simulink model "vertical_smm_3d_with_xz_lqr_with_torque_cmds"  (R2015a)
settings: Solver=FixedStepDiscrete  SolverMode=SingleTasking  StartTime=0.0  StopTime=inf  FixedStep=sample_time  RelTol=1e-3
values from neighbouring files (symbols this model uses):
  forward_dx_of_dxstar = [-1.33147741515 -1.28147741462 -1.23147741409 -1.18147741356 -1.13147741303 -1.0814774125 -1.03147741197 -0.981477411445 -0.931477410916 -0.881477410388 -0.831477409975 -0.781477409737 ... (28413 elements, 41x21x33)]    [ref_trajs.mat]
  forward_x_of_dxstar = [0.245075236011 0.237749717983 0.230424199955 0.223098681927 0.215773163898 0.20844764587 0.201122127842 0.193796609813 0.186471091785 0.179145573757 0.171820055745 0.164494537786 ... (28413 elements, 41x21x33)]    [ref_trajs.mat]
  target_dx_range = [-1 -0.95 -0.9 -0.85 -0.8 -0.75 -0.7 -0.65 -0.6 -0.55 -0.5 -0.45 ... (41 elements, 1x41)]    [ref_trajs.mat]
undefined symbols (not defined in the file or in its folder): A_kalman_fourbar_gear, A_kalman_transverse, A_kalman_vertical, A_lpf_accelerometer, A_lpf_dtau, A_lpf_fourbar_angles, A_lpf_imu, A_lpf_lateral_angle, A_lpf_leg_spring, B1_lpf_accelerometer, B1_lpf_dtau, B1_lpf_fourbar_angles, B1_lpf_imu, B1_lpf_lateral_angle, B1_lpf_leg_spring, B2_lpf_accelerometer, B2_lpf_dtau, B2_lpf_fourbar_angles, B2_lpf_imu, B2_lpf_lateral_angle, B2_lpf_leg_spring, B_dx_versus_x0, B_kalman_fourbar_gear, B_kalman_transverse, B_kalman_vertical, backwards_K_sag_of_t, backwards_P_sag_of_t, C_kalman_fourbar_gear, C_kalman_transverse, C_kalman_vertical, com_leg_motor, com_torso, contact_threshold, control_start_time, d_ankle_to_foot, d_vertical_com, desired_com_forward_velocity, desired_com_lateral_velocity, desired_initial_leg_roll_left, desired_initial_leg_roll_right, desired_stance_beta2, desired_standing_torso_pitch, desired_standing_torso_roll, desired_standing_z, desired_torso_pitch, desired_torso_roll, Discrete, enable_bouncing, enable_hopping, fcut_contact, g, HIP_MTR_MAX_CONT_TORQUE, HIP_MTR_MAX_TORQUE, i_leg_motor, i_robot, i_torso, initial_dx_estimate, initial_dy_estimate, initial_dz_estimate, initial_leg_selection ... (+77)
libraries: simulink x18, ctrlSharedLib x7
(part 2 of 5)

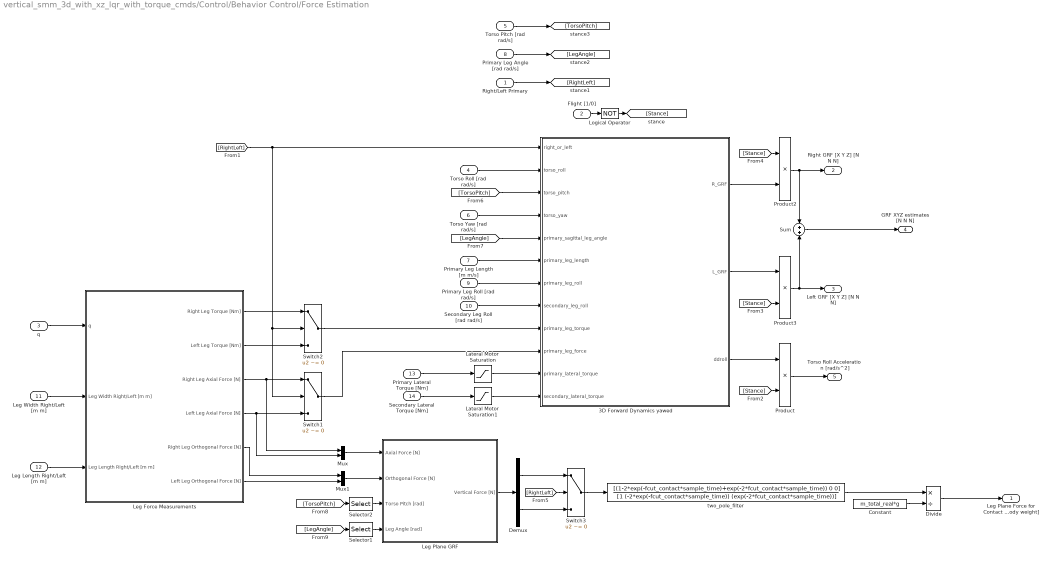
== system vertical_smm_3d_with_xz_lqr_with_torque_cmds/Control/Behavior Control/Force Estimation ==
  Right/Left Primary : Inport
  Flight [1/0] : Inport  Port=2
  q : Inport  Port=3
  Torso Roll [rad rad/s] : Inport  Port=4
  Torso Pitch [rad rad/s] : Inport  Port=5
  Torso Yaw [rad rad/s] : Inport  Port=6
  Primary Leg Length [m m/s] : Inport  Port=7
  Primary Leg Angle [rad rad/s] : Inport  Port=8
  Primary Leg Roll [rad rad/s] : Inport  Port=9
  Secondary Leg Roll [rad rad/s] : Inport  Port=10
  Leg Width Right/Left [m m] : Inport  Port=11
  Leg Length Right/Left [m m] : Inport  Port=12
  Primary Lateral Torque [Nm] : Inport  Port=13
  Secondary Lateral Torque [Nm] : Inport  Port=14
  3D Forward Dynamics yawed : MATLAB Function  TreatAsAtomicUnit=on
  Constant : Constant  Value=m_total_real*g
  Demux : Demux  Outputs=2
  Divide : Product  Inputs=*/
  Lateral Motor Saturation : Saturate  UpperLimit=HIP_MTR_MAX_TORQUE  LowerLimit=-HIP_MTR_MAX_TORQUE
      settings: AttributesFormatString=Top: %<UpperLimit>\nBottom: %<LowerLimit>
  Lateral Motor Saturation1 : Saturate  UpperLimit=HIP_MTR_MAX_TORQUE  LowerLimit=-HIP_MTR_MAX_TORQUE
      settings: AttributesFormatString=Top: %<UpperLimit>\nBottom: %<LowerLimit>
  Leg Force Measurements : Subsystem
  Leg Plane GRF : Subsystem
  Logical Operator : Logic  Operator=NOT  AllPortsSameDT=off  OutDataTypeStr=boolean
  Mux : Mux  Inputs=2
  Mux1 : Mux  Inputs=2
  Product : Product
  Product2 : Product
  Product3 : Product
  Selector1 : Selector  InputPortWidth=2  Indices=[1]
  Selector2 : Selector  InputPortWidth=2  Indices=[1]
  Sum : Sum  Inputs=+|+
  Switch1 : Switch  Criteria=u2 ~= 0
  Switch2 : Switch  Criteria=u2 ~= 0
  Switch3 : Switch  Criteria=u2 ~= 0
  two_pole_filter : DiscreteTransferFcn  Numerator=[(1-2*exp(-fcut_contact*sample_time)+exp(-2*fcut_contact*sample_time)) 0 0]  Denominator=[1 (-2*exp(-fcut_contact*sample_time)) (exp(-2*fcut_contact*sample_time))]  SampleTime=sample_time
  Leg Plane Force for Contact Detection [body weight] : Outport
  Right GRF [X Y Z] [N N N] : Outport  Port=2
  Left GRF [X Y Z] [N N N] : Outport  Port=3
  GRF XYZ estimates [N N N] : Outport  Port=4  OutputWhenDisabled=reset  InitialOutput=[0 0 0 0 0 0]
  Torso Roll Acceleration [rad/s^2] : Outport  Port=5  OutputWhenDisabled=reset  InitialOutput=[0 0 0 0 0 0]
  wires:
  Divide/1 -> Leg Plane Force for Contact Detection [body weight]/1
  Leg Width Right/Left [m m]/1 -> Leg Force Measurements/2(Leg Width Right/Left [m m])
  q/1 -> Leg Force Measurements/1(q)
  two_pole_filter/1 -> Divide/1
  Constant/1 -> Divide/2
  [RightLeft] -> 3D Forward Dynamics yawed/1(right_or_left), Switch2/2, Switch1/2
  Leg Length Right/Left [m m]/1 -> Leg Force Measurements/3(Leg Length Right/Left [m m])
  3D Forward Dynamics yawed/1(R_GRF) -> Product2/2
  3D Forward Dynamics yawed/2(L_GRF) -> Product3/1
  3D Forward Dynamics yawed/3(ddroll) -> Product/1
  Leg Force Measurements/3(Right Leg Axial Force [N]) -> Mux/1, Switch1/1
  Leg Force Measurements/4(Left Leg Axial Force [N]) -> Switch1/3, Mux/2
  Switch1/1 -> 3D Forward Dynamics yawed/10(primary_leg_force)
  [TorsoPitch] -> 3D Forward Dynamics yawed/3(torso_pitch)
  Torso Roll [rad rad/s]/1 -> 3D Forward Dynamics yawed/2(torso_roll)
  Torso Yaw [rad rad/s]/1 -> 3D Forward Dynamics yawed/4(torso_yaw)
  Primary Leg Length [m m/s]/1 -> 3D Forward Dynamics yawed/6(primary_leg_length)
  [LegAngle] -> 3D Forward Dynamics yawed/5(primary_sagittal_leg_angle)
  Flight [1/0]/1 -> Logical Operator/1
  [Stance] -> Product/2
  Product/1 -> Torso Roll Acceleration [rad/s^2]/1
  Switch3/1 -> two_pole_filter/1
  Logical Operator/1 -> [Stance]
  Product3/1 -> Left GRF [X Y Z] [N N N]/1, Sum/2
  Product2/1 -> Right GRF [X Y Z] [N N N]/1, Sum/1
  [Stance] -> Product3/2
  [Stance] -> Product2/1
  Primary Leg Roll [rad rad/s]/1 -> 3D Forward Dynamics yawed/7(primary_leg_roll)
  Secondary Leg Roll [rad rad/s]/1 -> 3D Forward Dynamics yawed/8(secondary_leg_roll)
  Switch2/1 -> 3D Forward Dynamics yawed/9(primary_leg_torque)
  Leg Force Measurements/1(Right Leg Torque [Nm]) -> Switch2/1
  Leg Force Measurements/2(Left Leg Torque [Nm]) -> Switch2/3
  Sum/1 -> GRF XYZ estimates [N N N]/1
  Mux1/1 -> Leg Plane GRF/2(Orthogonal Force [N])
  Mux/1 -> Leg Plane GRF/1(Axial Force [N])
  Leg Force Measurements/5(Right Leg Orthogonal Force [N]) -> Mux1/1
  Leg Force Measurements/6(Left Leg Orthogonal Force [N]) -> Mux1/2
  Right/Left Primary/1 -> [RightLeft]
  [RightLeft] -> Switch3/2
  Leg Plane GRF/1(Vertical Force [N]) -> Demux/1
  Demux/1 -> Switch3/1
  Demux/2 -> Switch3/3
  Primary Leg Angle [rad rad/s]/1 -> [LegAngle]
  Torso Pitch [rad rad/s]/1 -> [TorsoPitch]
  [LegAngle] -> Selector1/1
  Selector1/1 -> Leg Plane GRF/4(Leg Angle [rad])
  [TorsoPitch] -> Selector2/1
  Selector2/1 -> Leg Plane GRF/3(Torso Pitch [rad])
  Primary Lateral Torque [Nm]/1 -> Lateral Motor Saturation/1
  Secondary Lateral Torque [Nm]/1 -> Lateral Motor Saturation1/1
  Lateral Motor Saturation/1 -> 3D Forward Dynamics yawed/11(primary_lateral_torque)
  Lateral Motor Saturation1/1 -> 3D Forward Dynamics yawed/12(secondary_lateral_torque)

== system vertical_smm_3d_with_xz_lqr_with_torque_cmds/Control/Behavior Control/L Leg Calculator ==
  Front [rad rad/s] : Inport
  Back [rad rad/s] : Inport  Port=2
  Constant : Constant  Value=d_ankle_to_foot-0.01
  Demux1 : Demux  Outputs=2
  Gain1 : Gain  Gain=2*l_seg
  Gain2 : Gain  Gain=l_seg
  Gain3 : Gain  Gain=-1
  Gain4 : Gain  Gain=0.5
  Gain5 : Gain  Gain=0.5
  Gain6 : Gain  Gain=2
  Mux1 : Mux  Inputs=2
  Product : Product  RndMeth=Zero
  Sum : Sum  Inputs=++|
  Sum4 : Sum  Inputs=+|+
  Sum5 : Sum  Inputs=+|-
  Trigonometric Function : Trigonometry  Operator=cos
  Trigonometric Function1 : Trigonometry
  "Leg Length [m m/s] " : Outport
  Leg Angle [rad rad/s] : Outport  Port=2
  Leg Splay [rad rad/s] : Outport  Port=3
  w [m] : Outport  Port=4
  wires:
  Sum/1 -> Mux1/1
  Constant/1 -> Sum/1
  Sum4/1 -> Gain5/1
  Mux1/1 -> "Leg Length [m m/s] "/1
  Sum5/1 -> Demux1/1, Leg Splay [rad rad/s]/1
  Gain2/1 -> Gain6/1, Product/1
  Demux1/1 -> Gain4/1
  Gain3/1 -> Product/2
  Demux1/2 -> Gain3/1
  Back [rad rad/s]/1 -> Sum5/1, Sum4/1
  Front [rad rad/s]/1 -> Sum4/2, Sum5/2
  Product/1 -> Mux1/2
  Trigonometric Function1/1 -> Gain2/1
  Gain1/1 -> Sum/2
  Trigonometric Function/1 -> Gain1/1
  Gain4/1 -> Trigonometric Function/1, Trigonometric Function1/1
  Gain6/1 -> w [m]/1
  Gain5/1 -> Leg Angle [rad rad/s]/1

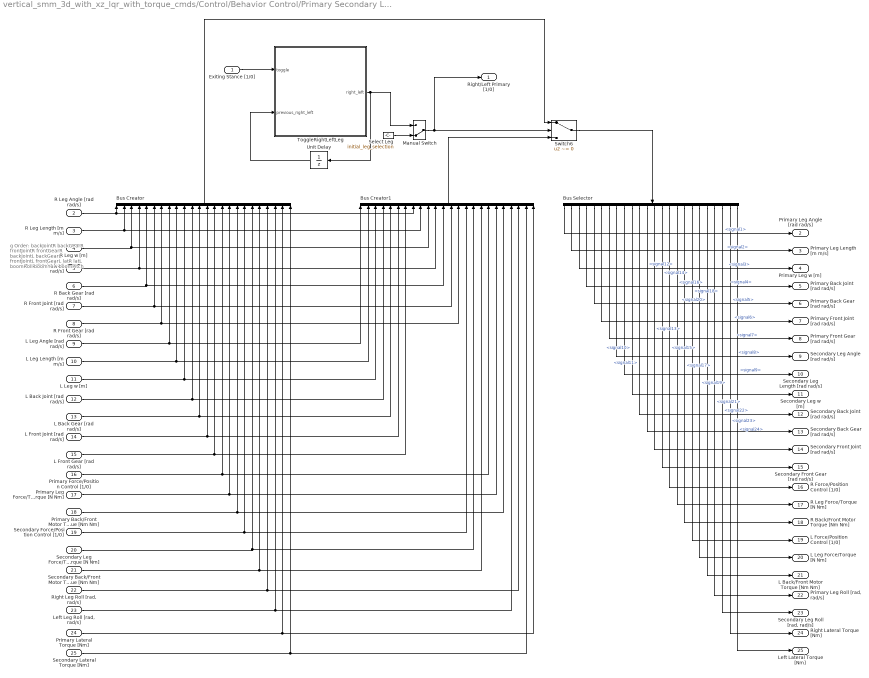
== system vertical_smm_3d_with_xz_lqr_with_torque_cmds/Control/Behavior Control/Primary Secondary Leg Swap ==
  note: q Order:
      |
      | backJointR
      | backGearR
      | frontJointR
      | frontGearR
      |
      | backJointL
      | backGearL
      | frontJointL
      | frontGearL
      |
      | latR
      | latL
      |
      | boomRoll
      | boomYaw
      | boomPitch
  Exiting Stance [1/0] : Inport
  R Leg Angle [rad rad/s] : Inport  Port=2
  R Leg Length [m m/s] : Inport  Port=3
  R Leg w [m] : Inport  Port=4
  R Back Joint [rad rad/s] : Inport  Port=5
  R Back Gear [rad rad/s] : Inport  Port=6
  R Front Joint [rad rad/s] : Inport  Port=7
  R Front Gear [rad rad/s] : Inport  Port=8
  L Leg Angle [rad rad/s] : Inport  Port=9
  L Leg Length [m m/s] : Inport  Port=10
  L Leg w [m] : Inport  Port=11
  L Back Joint [rad rad/s] : Inport  Port=12
  L Back Gear [rad rad/s] : Inport  Port=13
  L Front Joint [rad rad/s] : Inport  Port=14
  L Front Gear [rad rad/s] : Inport  Port=15
  Primary Force/Position Control [1/0] : Inport  Port=16
  Primary Leg Force/Torque [N Nm] : Inport  Port=17
  Primary Back/Front Motor Torque [Nm Nm] : Inport  Port=18
  Secondary Force/Position Control [1/0] : Inport  Port=19
  Secondary Leg Force/Torque [N Nm] : Inport  Port=20
  Secondary Back/Front Motor Torque [Nm Nm] : Inport  Port=21
  "Right Leg Roll [rad, rad/s]" : Inport  Port=22
  "Left Leg Roll [rad, rad/s]" : Inport  Port=23
  Primary Lateral Torque [Nm] : Inport  Port=24
  Secondary Lateral Torque [Nm] : Inport  Port=25
  Bus Creator : BusCreator  Inputs=24
  Bus Creator1 : BusCreator  Inputs=24
  Bus Selector : BusSelector  OutputSignals=signal1,signal2,signal3,signal4,signal5,signal6,signal7,signal8,signal9,signal10,signal11,signal12,signal13,signal14,signal15,signal16,signal17,signal18,signal19,signal20,signal21,signal22,signal23,signal24
  Manual Switch : ManualSwitch  CurrentSetting=0
  Select Leg : Constant  Value=initial_leg_selection  OutDataTypeStr=boolean
  Switch6 : Switch  Criteria=u2 ~= 0  OutDataTypeStr=Inherit: Inherit via back propagation  ZeroCross=off
  ToggleRightLeftLeg : MATLAB Function  TreatAsAtomicUnit=on
      settings: MinAlgLoopOccurrences=on
  Unit Delay : UnitDelay  InitialCondition=initial_leg_selection  SampleTime=sample_time
  Right/Left Primary [1/0] : Outport
  Primary Leg Angle [rad rad/s] : Outport  Port=2
  Primary Leg Length [m m/s] : Outport  Port=3
  Primary Leg w [m] : Outport  Port=4
  Primary Back Joint [rad rad/s] : Outport  Port=5
  Primary Back Gear [rad rad/s] : Outport  Port=6
  Primary Front Joint [rad rad/s] : Outport  Port=7
  Primary Front Gear [rad rad/s] : Outport  Port=8
  Secondary Leg Angle [rad rad/s] : Outport  Port=9
  Secondary Leg Length [rad rad/s] : Outport  Port=10
  Secondary Leg w [m] : Outport  Port=11
  Secondary Back Joint [rad rad/s] : Outport  Port=12
  Secondary Back Gear [rad rad/s] : Outport  Port=13
  Secondary Front Joint [rad rad/s] : Outport  Port=14
  Secondary Front Gear [rad rad/s] : Outport  Port=15
  R Force/Position Control [1/0] : Outport  Port=16
  R Leg Force/Torque [N Nm] : Outport  Port=17
  R Back/Front Motor Torque [Nm Nm] : Outport  Port=18
  L Force/Position Control [1/0] : Outport  Port=19
  L Leg Force/Torque [N Nm] : Outport  Port=20
  L Back/Front Motor Torque [Nm Nm] : Outport  Port=21
  "Primary Leg Roll [rad, rad/s]" : Outport  Port=22
  "Secondary Leg Roll [rad, rad/s]" : Outport  Port=23
  Right Lateral Torque [Nm] : Outport  Port=24
  Left Lateral Torque [Nm] : Outport  Port=25
  wires:
  Unit Delay/1 -> ToggleRightLeftLeg/2(previous_right_left)
  Exiting Stance [1/0]/1 -> ToggleRightLeftLeg/1(toggle)
  ToggleRightLeftLeg/1(right_left) -> Unit Delay/1, Manual Switch/1
  Manual Switch/1 -> Right/Left Primary [1/0]/1, Switch6/2
  Select Leg/1 -> Manual Switch/2
  R Leg w [m]/1 -> Bus Creator1/10, Bus Creator/3
  R Leg Angle [rad rad/s]/1 -> Bus Creator1/8, Bus Creator/1
  R Leg Length [m m/s]/1 -> Bus Creator1/9, Bus Creator/2
  Bus Creator/1 -> Switch6/1
  Bus Creator1/1 -> Switch6/3
  R Back Joint [rad rad/s]/1 -> Bus Creator1/11, Bus Creator/4
  R Back Gear [rad rad/s]/1 -> Bus Creator1/12, Bus Creator/5
  R Front Joint [rad rad/s]/1 -> Bus Creator1/13, Bus Creator/6
  R Front Gear [rad rad/s]/1 -> Bus Creator1/14, Bus Creator/7
  L Leg Angle [rad rad/s]/1 -> Bus Creator1/1, Bus Creator/8
  L Leg Length [m m/s]/1 -> Bus Creator1/2, Bus Creator/9
  L Leg w [m]/1 -> Bus Creator1/3, Bus Creator/10
  L Back Joint [rad rad/s]/1 -> Bus Creator1/4, Bus Creator/11
  L Back Gear [rad rad/s]/1 -> Bus Creator1/5, Bus Creator/12
  L Front Joint [rad rad/s]/1 -> Bus Creator/13, Bus Creator1/6
  L Front Gear [rad rad/s]/1 -> Bus Creator1/7, Bus Creator/14
  Primary Force/Position Control [1/0]/1 -> Bus Creator1/18, Bus Creator/15
  Primary Leg Force/Torque [N Nm]/1 -> Bus Creator1/19, Bus Creator/16
  Primary Back/Front Motor Torque [Nm Nm]/1 -> Bus Creator1/20, Bus Creator/17
  Secondary Force/Position Control [1/0]/1 -> Bus Creator1/15, Bus Creator/18
  Secondary Leg Force/Torque [N Nm]/1 -> Bus Creator1/16, Bus Creator/19
  Secondary Back/Front Motor Torque [Nm Nm]/1 -> Bus Creator1/17, Bus Creator/20
  Switch6/1 -> Bus Selector/1
  Bus Selector/1 -> Primary Leg Angle [rad rad/s]/1  "<signal1>"
  Bus Selector/2 -> Primary Leg Length [m m/s]/1  "<signal2>"
  Bus Selector/3 -> Primary Leg w [m]/1  "<signal3>"
  Bus Selector/4 -> Primary Back Joint [rad rad/s]/1  "<signal4>"
  Bus Selector/5 -> Primary Back Gear [rad rad/s]/1  "<signal5>"
  Bus Selector/6 -> Primary Front Joint [rad rad/s]/1  "<signal6>"
  Bus Selector/7 -> Primary Front Gear [rad rad/s]/1  "<signal7>"
  Bus Selector/8 -> Secondary Leg Angle [rad rad/s]/1  "<signal8>"
  Bus Selector/9 -> Secondary Leg Length [rad rad/s]/1  "<signal9>"
  Bus Selector/10 -> Secondary Leg w [m]/1  "<signal10>"
  Bus Selector/11 -> Secondary Back Joint [rad rad/s]/1  "<signal11>"
  Bus Selector/12 -> Secondary Back Gear [rad rad/s]/1  "<signal12>"
  Bus Selector/13 -> Secondary Front Joint [rad rad/s]/1  "<signal13>"
  Bus Selector/14 -> Secondary Front Gear [rad rad/s]/1  "<signal14>"
  Bus Selector/15 -> R Force/Position Control [1/0]/1  "<signal15>"
  Bus Selector/16 -> R Leg Force/Torque [N Nm]/1  "<signal16>"
  Bus Selector/17 -> R Back/Front Motor Torque [Nm Nm]/1  "<signal17>"
  Bus Selector/18 -> L Force/Position Control [1/0]/1  "<signal18>"
  Bus Selector/19 -> L Leg Force/Torque [N Nm]/1  "<signal19>"
  Bus Selector/20 -> L Back/Front Motor Torque [Nm Nm]/1  "<signal20>"
  "Right Leg Roll [rad, rad/s]"/1 -> Bus Creator1/22, Bus Creator/21
  "Left Leg Roll [rad, rad/s]"/1 -> Bus Creator1/21, Bus Creator/22
  Bus Selector/21 -> "Primary Leg Roll [rad, rad/s]"/1  "<signal21>"
  Bus Selector/22 -> "Secondary Leg Roll [rad, rad/s]"/1  "<signal22>"
  Primary Lateral Torque [Nm]/1 -> Bus Creator1/24, Bus Creator/23
  Secondary Lateral Torque [Nm]/1 -> Bus Creator1/23, Bus Creator/24
  Bus Selector/23 -> Right Lateral Torque [Nm]/1  "<signal23>"
  Bus Selector/24 -> Left Lateral Torque [Nm]/1  "<signal24>"

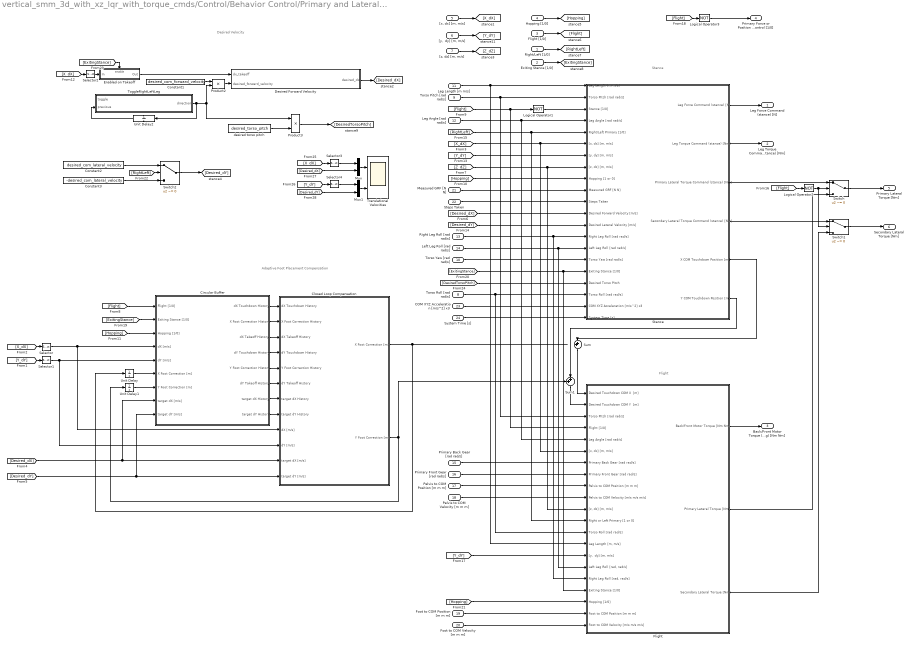
== system vertical_smm_3d_with_xz_lqr_with_torque_cmds/Control/Behavior Control/Primary and Lateral Behavior ==
  note: Stance
  note: Flight
  note: Adaptive Foot Placement Compensation
  note: Desired Velocity
  Right/Left [1/0] : Inport
  Exiting Stance [1/0] : Inport  Port=2
  Flight [1/0] : Inport  Port=3
  Hopping [1/0] : Inport  Port=4
  "[x, dx] [m, m/s]" : Inport  Port=5
  "[y,  dy] [m, m/s]" : Inport  Port=6
  "[z, dz] [m, m/s]" : Inport  Port=7
  Torso Roll [rad rad/s] : Inport  Port=8
  Torso Pitch [rad rad/s] : Inport  Port=9
  Torso Yaw [rad rad/s] : Inport  Port=10
  Leg Length [m m/s] : Inport  Port=11
  Leg Angle [rad rad/s] : Inport  Port=12
  Right Leg Roll [rad rad/s] : Inport  Port=13
  Left Leg Roll [rad rad/s] : Inport  Port=14
  Primary Back Gear [rad rad/s] : Inport  Port=15
  Primary Front Gear [rad rad/s] : Inport  Port=16
  Pelvis to COM Position [m m m] : Inport  Port=17
  Pelvis to COM Velocity [m m m] : Inport  Port=18
  Foot to COM Position [m m m] : Inport  Port=19
  Foot to COM Velocity [m m m] : Inport  Port=20
  Measured GRF [N N] : Inport  Port=21
  Steps Taken : Inport  Port=22
  COM XYZ Acceleration [m/s^2] x3 : Inport  Port=23
  System Time [s] : Inport  Port=24
  Circular Buffer : Subsystem
  Closed Loop Compensation : Subsystem
  Constant1 : Constant  Value=desired_com_forward_velocity
  Constant2 : Constant  Value=desired_com_lateral_velocity
  Constant3 : Constant  Value=-desired_com_lateral_velocity
  Desired Forward Velocity : MATLAB Function  TreatAsAtomicUnit=on
  Enabled on Takeoff : Subsystem  TreatAsAtomicUnit=on
  Flight : Subsystem
  Logical Operator1 : Logic  Operator=NOT  AllPortsSameDT=off  OutDataTypeStr=boolean
  Logical Operator2 : Logic  Operator=NOT  AllPortsSameDT=off  OutDataTypeStr=boolean
  Logical Operator3 : Logic  Operator=NOT  AllPortsSameDT=off  OutDataTypeStr=boolean
  Mux : Mux  Inputs=2
  Mux1 : Mux  Inputs=2
  Product2 : Product
  Product3 : Product
  Selector{,1..4} (5 alike) : Selector  InputPortWidth=2  Indices=[2]
  Stance : Subsystem
  Sum : Sum  Inputs=++|
  Sum1 : Sum  Inputs=++|
  Switch : Switch  Criteria=u2 ~= 0
  Switch1 : Switch  Criteria=u2 ~= 0
  Switch2 : Switch  Criteria=u2 ~= 0
  ToggleRightLeftLeg : MATLAB Function  TreatAsAtomicUnit=on
      settings: MinAlgLoopOccurrences=on
  Translational Velocities : Scope  NumInputPorts=2
      settings: YMin=-1000~-5  YMax=1000~5  SaveName=ScopeData2  SampleInput=on
  Unit Delay : UnitDelay  SampleTime=-1
  Unit Delay1 : UnitDelay  SampleTime=-1
  Unit Delay2 : UnitDelay  InitialCondition=1  SampleTime=sample_time
  desired torso pitch : Constant  Value=desired_torso_pitch
  Leg Force Command (stance) [N] : Outport
  Leg Torque Command (stance) [Nm] : Outport  Port=2
  Back/Front Motor Torque (swing) [Nm Nm] : Outport  Port=3
  Primary Force or Position Control [1/0] : Outport  Port=4  OutDataTypeStr=boolean
  Primary Lateral Torque [Nm] : Outport  Port=5
  Secondary Lateral Torque [Nm] : Outport  Port=6
  wires:
  Leg Length [m m/s]/1 -> Stance/1(Leg Length [m m/s]), Flight/14("Leg Length [m, m/s]")
  Stance/1(Leg Force Command (stance) [N]) -> Leg Force Command (stance) [N]/1
  Stance/2(Leg Torque Command (stance) [Nm]) -> Leg Torque Command (stance) [Nm]/1
  Torso Pitch [rad rad/s]/1 -> Stance/2(Torso Pitch [rad rad/s]), Flight/3(Torso Pitch [rad rad/s])
  [Hopping] -> Stance/9(Hopping [1 or 0])
  [X_dX] -> Stance/6("[x, dx] [m, m/s]"), Flight/6("[x, dx] [m, m/s]")
  [RightLeft] -> Stance/5(Right/Left Primary [1/0]), Flight/12(Right or Left Primary [1 or 0])
  Primary Back Gear [rad rad/s]/1 -> Flight/7(Primary Back Gear [rad rad/s])
  Primary Front Gear [rad rad/s]/1 -> Flight/8(Primary Front Gear [rad rad/s])
  Leg Angle [rad rad/s]/1 -> Stance/4(Leg Angle [rad rad/s]), Flight/5(Leg Angle [rad rad/s])
  Flight/1(Back/Front Motor Torque [Nm Nm]) -> Back/Front Motor Torque (swing) [Nm Nm]/1
  Logical Operator1/1 -> Stance/3(Stance [1/0])
  [Flight] -> Circular Buffer/1(Flight [1/0])
  Pelvis to COM Position [m m m]/1 -> Flight/9(Pelvis to COM Position [m m m])
  [Z_dZ] -> Stance/8("[z, dz] [m, m/s]"), Flight/11("[z, dz] [m, m/s]")
  Pelvis to COM Velocity [m m m]/1 -> Flight/10(Pelvis to COM Velocity [m/s m/s m/s])
  Torso Roll [rad rad/s]/1 -> Stance/19(Torso Roll [rad rad/s]), Flight/13(Torso Roll [rad rad/s])
  Measured GRF [N N]/1 -> Stance/10(Measured GRF [N N])
  Steps Taken/1 -> Stance/11(Steps Taken)
  [Y_dY] -> Flight/15("[y,  dy] [m, m/s]")
  Circular Buffer/1("dX Touchdown History ") -> Closed Loop Compensation/1(dX Touchdown History)
  Circular Buffer/2(X Foot Correction History) -> Closed Loop Compensation/2(X Foot Correction History)
  Circular Buffer/3(dX Takeoff History) -> Closed Loop Compensation/3(dX Takeoff History)
  Circular Buffer/4("dY Touchdown History ") -> Closed Loop Compensation/4(dY Touchdown History)
  Circular Buffer/5(Y Foot Correction History) -> Closed Loop Compensation/5(Y Foot Correction History)
  Circular Buffer/6(dY Takeoff History) -> Closed Loop Compensation/6(dY Takeoff History)
  Circular Buffer/8(target dY History) -> Closed Loop Compensation/8(target dY History)
  Circular Buffer/7(target dX History) -> Closed Loop Compensation/7(target dX History)
  [Desired_dX] -> Circular Buffer/8(target dX [m/s]), Closed Loop Compensation/11(target dX [m/s])
  [Desired_dY] -> Circular Buffer/9(target dY [m/s]), Closed Loop Compensation/12("target dY [m/s] ")
  Stance/5(X COM Touchdown Position [m]) -> Sum/2
  Sum/1 -> Flight/1(Desired Touchdown COM X  [m])
  Closed Loop Compensation/1(X Foot Correction [m]) -> Unit Delay/1
  Selector1/1 -> Circular Buffer/5(dY [m/s]), Closed Loop Compensation/10(dY [m/s])
  Selector/1 -> Circular Buffer/4(dX [m/s]), Closed Loop Compensation/9(dX [m/s])
  Unit Delay1/1 -> Circular Buffer/7(Y Foot Correction [m])
  Unit Delay/1 -> Circular Buffer/6(X Foot Correction [m])
  Closed Loop Compensation/2(Y Foot Correction [m]) -> Unit Delay1/1, Sum1/1
  "[x, dx] [m, m/s]"/1 -> [X_dX]
  "[z, dz] [m, m/s]"/1 -> [Z_dZ]
  "[y,  dy] [m, m/s]"/1 -> [Y_dY]
  [X_dX] -> Selector/1
  [Y_dY] -> Selector1/1
  [Desired_dX] -> Stance/12(Desired Forward Velocity [m/s])
  Flight [1/0]/1 -> [Flight]
  [Flight] -> Flight/4(Flight [1/0]), Logical Operator1/1
  Hopping [1/0]/1 -> [Hopping]
  Stance/6(Y COM Touchdown Position [m]) -> Sum1/2
  Sum1/1 -> Flight/2(Desired Touchdown COM Y  [m])
  Right Leg Roll [rad rad/s]/1 -> Stance/14(Right Leg Roll [rad rad/s]), Flight/17("Right Leg Roll [rad, rad/s]")
  Left Leg Roll [rad rad/s]/1 -> Stance/15(Left Leg Roll [rad rad/s]), Flight/16("Left Leg Roll [rad, rad/s]")
  [Y_dY] -> Stance/7("[y, dy] [m, m/s]")
  [Desired_dY] -> Stance/13(Desired Lateral Velocity [m/s])
  Right/Left [1/0]/1 -> [RightLeft]
  Logical Operator2/1 -> Switch1/2, Switch/2
  Stance/3(Primary Lateral Torque Command (stance) [Nm]) -> Switch/1
  Flight/2(Primary Lateral Torque [Nm]) -> Switch/3
  Stance/4(Secondary Lateral Torque Command (stance) [Nm]) -> Switch1/1
  Flight/3(Secondary Lateral Torque [Nm]) -> Switch1/3
  [Flight] -> Logical Operator2/1
  Switch/1 -> Primary Lateral Torque [Nm]/1
  Switch1/1 -> Secondary Lateral Torque [Nm]/1
  [Flight] -> Logical Operator3/1
  Logical Operator3/1 -> Primary Force or Position Control [1/0]/1
  Torso Yaw [rad rad/s]/1 -> Stance/16(Torso Yaw [rad rad/s])
  [Hopping] -> Circular Buffer/3(Hopping [1/0])
  [ExitingStance] -> Circular Buffer/2(Exiting Stance [1/0])
  Exiting Stance [1/0]/1 -> [ExitingStance]
  [ExitingStance] -> Stance/17(Exiting Stance [1/0]), Flight/18(Exiting Stance [1/0])
  [Hopping] -> Flight/19(Hopping [1/0])
  [X_dX] -> Selector2/1
  Switch2/1 -> [Desired_dY]
  Enabled on Takeoff/1(Out) -> Desired Forward Velocity/1(dx_takeoff)
  [RightLeft] -> Switch2/2
  Constant2/1 -> Switch2/1
  Constant3/1 -> Switch2/3
  [ExitingStance] -> Enabled on Takeoff/Enable
  Selector2/1 -> Enabled on Takeoff/1(In)
  Desired Forward Velocity/1(desired_dx) -> [Desired_dX]
  Product2/1 -> Desired Forward Velocity/2(desired_forward_velocity)
  ToggleRightLeftLeg/1(direction) -> Product2/2, Product3/1, Unit Delay2/1
  Unit Delay2/1 -> ToggleRightLeftLeg/2(previous)
  Constant1/1 -> Product2/1
  desired torso pitch/1 -> Product3/2
  Product3/1 -> [DesiredTorsoPitch]
  [DesiredTorsoPitch] -> Stance/18(Desired Torso Pitch)
  Foot to COM Position [m m m]/1 -> Flight/20(Foot to COM Position [m m m])
  Foot to COM Velocity [m m m]/1 -> Flight/21(Foot to COM Velocity [m/s m/s m/s])
  [X_dX] -> Selector3/1
  Selector3/1 -> Mux/1
  [Y_dY] -> Selector4/1
  Selector4/1 -> Mux1/1
  Mux/1 -> Translational Velocities/1
  Mux1/1 -> Translational Velocities/2
  [Desired_dY] -> Mux1/2
  [Desired_dX] -> Mux/2
  COM XYZ Acceleration [m/s^2] x3/1 -> Stance/20(COM XYZ Acceleration [m/s^2] x3)
  System Time [s]/1 -> Stance/21(System Time [s])

== system vertical_smm_3d_with_xz_lqr_with_torque_cmds/Control/Behavior Control/R Leg Calculator ==
  Front [rad rad/s] : Inport
  Back [rad rad/s] : Inport  Port=2
  Constant : Constant  Value=d_ankle_to_foot-0.01
  Demux1 : Demux  Outputs=2
  Gain1 : Gain  Gain=2*l_seg
  Gain2 : Gain  Gain=l_seg
  Gain3 : Gain  Gain=-1
  Gain4 : Gain  Gain=0.5
  Gain5 : Gain  Gain=0.5
  Gain6 : Gain  Gain=2
  Mux1 : Mux  Inputs=2
  Product : Product  RndMeth=Zero
  Sum : Sum  Inputs=++|
  Sum4 : Sum  Inputs=+|+
  Sum5 : Sum  Inputs=+|-
  Trigonometric Function : Trigonometry  Operator=cos
  Trigonometric Function1 : Trigonometry
  "Leg Length [m m/s] " : Outport
  Leg Angle [rad rad/s] : Outport  Port=2
  Leg Splay [rad rad/s] : Outport  Port=3
  w [m] : Outport  Port=4
  wires:
  Constant/1 -> Sum/1
  Sum/1 -> Mux1/1
  Gain6/1 -> w [m]/1
  Gain4/1 -> Trigonometric Function1/1, Trigonometric Function/1
  Trigonometric Function/1 -> Gain1/1
  Gain1/1 -> Sum/2
  Trigonometric Function1/1 -> Gain2/1
  Product/1 -> Mux1/2
  Front [rad rad/s]/1 -> Sum5/2, Sum4/2
  Back [rad rad/s]/1 -> Sum4/1, Sum5/1
  Demux1/2 -> Gain3/1
  Gain3/1 -> Product/2
  Demux1/1 -> Gain4/1
  Gain2/1 -> Product/1, Gain6/1
  Sum5/1 -> Leg Splay [rad rad/s]/1, Demux1/1
  Mux1/1 -> "Leg Length [m m/s] "/1
  Sum4/1 -> Gain5/1
  Gain5/1 -> Leg Angle [rad rad/s]/1

== system vertical_smm_3d_with_xz_lqr_with_torque_cmds/Control/Behavior Control/Secondary Leg Behavior ==
  note: Mirror the primary
      | leg motion
  note: Position control the
      | individual four bar segments
  note: Convert to
      | four-bar angles
  Secondary Back Gear [rad rad/s] : Inport
  Secondary Front Gear [rad rad/s] : Inport  Port=2
  Torso Pitch [rad rad/s] : Inport  Port=3
  Right/Left Secondary [1/0] : Inport  Port=4
  Primary Leg Angle [rad rad/s] : Inport  Port=5
  Primary Leg Length [m m/s] : Inport  Port=6
  Avoid Hitting Mechanical Limits : MATLAB Function  TreatAsAtomicUnit=on
  Back/Front Motor PD : Subsystem
  Constant4 : Constant  Value=0
  Constant5 : Constant  Value=0  OutDataTypeStr=boolean
  Demux{1..3,5} (4 alike) : Demux  Outputs=2
  Demux6 : Demux  Outputs=6
  Fcn2 : Fcn  Expr=2*pi-u(1)
  Mirrored Leg Length Target : MATLAB Function  TreatAsAtomicUnit=on
  Mux{1..4,7,11} (6 alike) : Mux  Inputs=2
  Mux5 : Mux  Inputs=3
  Mux6 : Mux  Inputs=3
  Sum : Sum  Inputs=++|
  Virtual Leg to Four Bar : MATLAB Function  TreatAsAtomicUnit=on
  k_virtual1 : Gain  Gain=2
  k_virtual6 : Gain  Gain=-1
  two_pole_filter : DiscreteTransferFcn  Numerator=[A_lpf_leg_spring 0 0]  Denominator=[1 B1_lpf_leg_spring B2_lpf_leg_spring]  InitialStates=[pi, 0; pi, 0]*120.34  SampleTime=sample_time
  Secondary Back/Front Motor Torque [Nm Nm] : Outport
  Secondary Force or Position Control [1/0] : Outport  Port=2
  wires:
  Constant5/1 -> Secondary Force or Position Control [1/0]/1
  Demux5/2 -> k_virtual6/1
  Demux5/1 -> Fcn2/1
  Primary Leg Angle [rad rad/s]/1 -> two_pole_filter/1
  Mirrored Leg Length Target/2(dl_leg) -> Mux5/2
  Mirrored Leg Length Target/3(ddl_leg) -> Mux5/3
  Mirrored Leg Length Target/1(l_leg) -> Mux5/1
  Constant4/1 -> Mux6/3
  k_virtual6/1 -> Mux6/2
  Fcn2/1 -> Mux6/1
  Mux7/1 -> Demux6/1
  Mux5/1 -> Mux7/1
  Mux6/1 -> Mux7/2
  Virtual Leg to Four Bar/1(back) -> Avoid Hitting Mechanical Limits/1(back_desired)
  Virtual Leg to Four Bar/2(dback) -> Avoid Hitting Mechanical Limits/2(dback_desired)
  Virtual Leg to Four Bar/3(ddback) -> Avoid Hitting Mechanical Limits/3(ddback_desired)
  Virtual Leg to Four Bar/4(front) -> Avoid Hitting Mechanical Limits/4(front_desired)
  Virtual Leg to Four Bar/5(dfront) -> Avoid Hitting Mechanical Limits/5(dfront_desired)
  Virtual Leg to Four Bar/6(ddfront) -> Avoid Hitting Mechanical Limits/6(ddfront_desired)
  Demux6/1 -> Virtual Leg to Four Bar/1(l_leg)
  Demux6/2 -> Virtual Leg to Four Bar/2(dl_leg)
  Demux6/3 -> Virtual Leg to Four Bar/3(ddl_leg)
  Demux6/4 -> Virtual Leg to Four Bar/4(phi)
  Demux6/5 -> Virtual Leg to Four Bar/5(dphi)
  Demux6/6 -> Virtual Leg to Four Bar/6(ddphi)
  Mux11/1 -> Back/Front Motor PD/5(Measured Velocity [rad/s] [back front])
  Demux2/2 -> Mux11/2
  Mux4/1 -> Back/Front Motor PD/4(Measured Position [rad] [back front])
  Mux1/1 -> Back/Front Motor PD/1(Desired Position [rad] [back front])
  Right/Left Secondary [1/0]/1 -> Back/Front Motor PD/6(Right/Left Leg [1/0])
  Demux3/2 -> Mux11/1
  Demux3/1 -> Mux4/1
  Avoid Hitting Mechanical Limits/2(front_cmd) -> Mux1/2
  Avoid Hitting Mechanical Limits/1(back_cmd) -> Mux1/1
  Demux2/1 -> Mux4/2
  Secondary Front Gear [rad rad/s]/1 -> Demux2/1
  Secondary Back Gear [rad rad/s]/1 -> Demux3/1
  Avoid Hitting Mechanical Limits/3(dback_cmd) -> Mux2/1
  Avoid Hitting Mechanical Limits/4(dfront_cmd) -> Mux2/2
  Avoid Hitting Mechanical Limits/5(ddback_cmd) -> Mux3/1
  Avoid Hitting Mechanical Limits/6(ddfront_cmd) -> Mux3/2
  Mux2/1 -> Back/Front Motor PD/2(Desired Velocity [rad/s] [back front])
  Mux3/1 -> Back/Front Motor PD/3(Desired Acceleration [rad/s^2] [back front])
  two_pole_filter/1 -> Sum/2
  Demux1/1 -> Mirrored Leg Length Target/1(primary_l_leg)
  Demux1/2 -> Mirrored Leg Length Target/2(primary_dl_leg)
  Primary Leg Length [m m/s]/1 -> Demux1/1
  Back/Front Motor PD/1(Commanded Torque [Nm] [back front]) -> Secondary Back/Front Motor Torque [Nm Nm]/1
  Sum/1 -> Demux5/1
  Torso Pitch [rad rad/s]/1 -> k_virtual1/1
  k_virtual1/1 -> Sum/1

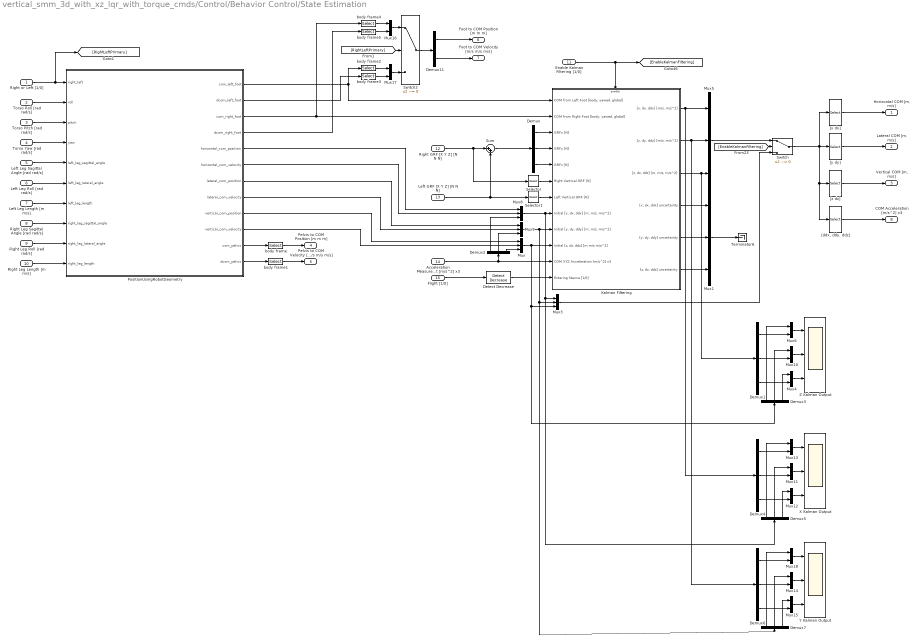
== system vertical_smm_3d_with_xz_lqr_with_torque_cmds/Control/Behavior Control/State Estimation ==
  Right or Left [1/0] : Inport
  Torso Roll [rad rad/s] : Inport  Port=2
  Torso Pitch [rad rad/s] : Inport  Port=3
  Torso Yaw [rad rad/s] : Inport  Port=4
  Left Leg Sagittal Angle [rad rad/s] : Inport  Port=5
  Left Leg Roll [rad rad/s] : Inport  Port=6
  Left Leg Length [m m/s] : Inport  Port=7
  Right Leg Sagittal Angle [rad rad/s] : Inport  Port=8
  Right Leg Roll [rad rad/s] : Inport  Port=9
  Right Leg Length [m m/s] : Inport  Port=10
  Enable Kalman Filtering [1/0] : Inport  Port=11
  Right GRF [X Y Z] [N N N] : Inport  Port=12
  Left GRF [X Y Z] [N N N] : Inport  Port=13
  " Acceleration Measurement [m/s^2] x3" : Inport  Port=14
  Flight [1/0] : Inport  Port=15
  Demux{,1..7} (8 alike) : Demux  Outputs=3
  Demux11 : Demux  Outputs=2
  Detect Decrease : simulink/Logic and Bit Operations/Detect Decrease  vinit=0.0  InputProcessing=Inherited  OutDataTypeStr=boolean
  Kalman Filtering : Subsystem
  Mux{,1,3,5,8..9} (6 alike) : Mux  Inputs=3
  Mux{4,6,10..18} (11 alike) : Mux  Inputs=2
  PositionUsingRobotGeometry : MATLAB Function  TreatAsAtomicUnit=on
  Selector : Selector  InputPortWidth=3  Indices=[3]
  Selector1 : Selector  InputPortWidth=3  Indices=[3]
  Sum : Sum  Inputs=|++
  Switch : Switch  Criteria=u2 ~= 0
  Switch2 : Switch  Criteria=u2 ~= 0
  Terminator6 : Terminator
  X Kalman Output : Scope  NumInputPorts=3
      settings: TimeRange=3.169818129988598  YMin=-0.035~-0.2~-1.75  YMax=0.015~0.225~2.25  SaveName=ScopeData29  SampleInput=on
  Y Kalman Output : Scope  NumInputPorts=3
      settings: TimeRange=39.999  YMin=0.05~-0.7~-2  YMax=0.18~1.1~3.5  SaveName=ScopeData30  SampleInput=on
  Z Kalman Output : Scope  NumInputPorts=3
      settings: TimeRange=3.175000000000004  YMin=0.865~-0.225~-1.2  YMax=0.96~0.225~1.2  SaveName=ScopeData27  SampleInput=on
  "[ddx, ddy, ddz]" : Selector  InputPortWidth=9  Indices=[3 6 9]
  "[x dx]" : Selector  InputPortWidth=9  Indices=[1 2]
  "[y dy]" : Selector  InputPortWidth=9  Indices=[4 5]
  "[z dz]" : Selector  InputPortWidth=9  Indices=[7 8]
  body frame : Selector  InputPortWidth=9  Indices=[1 2 3]
  body frame1 : Selector  InputPortWidth=9  Indices=[1 2 3]
  body frame{2..5} (4 alike) : Selector  InputPortWidth=9  Indices=[4 5 6]
  "Horizontal COM [m, m/s]" : Outport
  "Lateral COM [m, m/s]" : Outport  Port=2
  "Vertical COM [m, m/s]" : Outport  Port=3
  Pelvis to COM Position [m m m] : Outport  Port=4
  Pelvis to COM Velocity [m/s m/s m/s] : Outport  Port=5
  Foot to COM Position [m m m] : Outport  Port=6
  Foot to COM Velocity [m/s m/s m/s] : Outport  Port=7
  COM Acceleration [m/s^2] x3 : Outport  Port=8
  wires:
  Demux7/3 -> Mux15/1
  Demux7/2 -> Mux14/1
  Demux7/1 -> Mux18/1
  Demux6/3 -> Mux15/2
  Mux14/1 -> Y Kalman Output/2
  Demux6/1 -> Mux18/2
  Demux6/2 -> Mux14/2
  Mux18/1 -> Y Kalman Output/1
  Mux15/1 -> Y Kalman Output/3
  Demux5/3 -> Mux12/1
  Demux5/2 -> Mux11/1
  Demux5/1 -> Mux13/1
  Demux4/3 -> Mux12/2
  Mux11/1 -> X Kalman Output/2
  Demux4/1 -> Mux13/2
  Demux4/2 -> Mux11/2
  Mux13/1 -> X Kalman Output/1
  Mux12/1 -> X Kalman Output/3
  Demux3/3 -> Mux4/1
  Demux3/2 -> Mux10/1
  Demux3/1 -> Mux6/1
  Demux1/3 -> Mux4/2
  Mux10/1 -> Z Kalman Output/2
  Demux1/1 -> Mux6/2
  Demux1/2 -> Mux10/2
  Mux6/1 -> Z Kalman Output/1
  Mux4/1 -> Z Kalman Output/3
  Detect Decrease/1 -> Kalman Filtering/12(Entering Stance [1/0])
  Flight [1/0]/1 -> Detect Decrease/1
  body frame4/1 -> Mux16/1
  body frame5/1 -> Mux16/2
  body frame3/1 -> Mux17/2
  body frame2/1 -> Mux17/1
  Demux11/1 -> Foot to COM Position [m m m]/1
  Demux11/2 -> Foot to COM Velocity [m/s m/s m/s]/1
  Switch2/1 -> Demux11/1
  Mux16/1 -> Switch2/1
  Mux17/1 -> Switch2/3
  [RightLeftPrimary] -> Switch2/2
  PositionUsingRobotGeometry/6(horizontal_com_velocity) -> Mux8/2
  PositionUsingRobotGeometry/8(lateral_com_velocity) -> Mux9/2
  Mux/1 -> Kalman Filtering/10("Initial [z, dz, ddz] [m m/s m/s^2]"), Demux3/1, Mux3/3
  PositionUsingRobotGeometry/10(vertical_com_velocity) -> Mux/2
  PositionUsingRobotGeometry/9(vertical_com_position) -> Mux/1
  [EnableKalmanFiltering] -> Switch/2
  Kalman Filtering/6("[z, dz, ddz] uncertainty") -> Mux1/3
  Kalman Filtering/4("[x, dx, ddx] uncertainty") -> Mux1/1
  Kalman Filtering/5("[y, dy, ddy] uncertainty") -> Mux1/2
  Kalman Filtering/2("[y, dy, ddy] [m/s, m/s^2]") -> Mux5/2, Demux6/1
  Kalman Filtering/3("[z, dz, ddz] [m, m/s, m/s^2]") -> Mux5/3, Demux1/1
  Kalman Filtering/1("[x, dx, ddx] [m/s, m/s^2]") -> Mux5/1, Demux4/1
  Demux/2 -> Kalman Filtering/4(GRFy [N])
  Demux/3 -> Kalman Filtering/5(GRFz [N])
  "[y dy]"/1 -> "Lateral COM [m, m/s]"/1
  Switch/1 -> "[ddx, ddy, ddz]"/1, "[z dz]"/1, "[y dy]"/1, "[x dx]"/1
  "[z dz]"/1 -> "Vertical COM [m, m/s]"/1
  PositionUsingRobotGeometry/7(lateral_com_position) -> Mux9/1
  body frame1/1 -> Pelvis to COM Velocity [m/s m/s m/s]/1
  body frame/1 -> Pelvis to COM Position [m m m]/1
  "[x dx]"/1 -> "Horizontal COM [m, m/s]"/1
  PositionUsingRobotGeometry/11(com_pelvis) -> body frame/1
  PositionUsingRobotGeometry/12(dcom_pelvis) -> body frame1/1
  Mux1/1 -> Terminator6/1
  Demux/1 -> Kalman Filtering/3(GRFx [N])
  Enable Kalman Filtering [1/0]/1 -> [EnableKalmanFiltering], Kalman Filtering/Enable
  Sum/1 -> Demux/1
  Right GRF [X Y Z] [N N N]/1 -> Sum/1, Selector/1
  Left GRF [X Y Z] [N N N]/1 -> Sum/2, Selector1/1
  Selector1/1 -> Kalman Filtering/7(Left Vertical GRF [N])
  Selector/1 -> Kalman Filtering/6(Right Vertical GRF [N])
  Mux5/1 -> Switch/1
  PositionUsingRobotGeometry/4(dcom_right_foot) -> body frame5/1
  PositionUsingRobotGeometry/3(com_right_foot) -> Kalman Filtering/2("COM from Right Foot [body, yawed, global]"), body frame4/1
  PositionUsingRobotGeometry/2(dcom_left_foot) -> body frame3/1
  PositionUsingRobotGeometry/1(com_left_foot) -> Kalman Filtering/1("COM from Left Foot [body, yawed, global]"), body frame2/1
  Torso Pitch [rad rad/s]/1 -> PositionUsingRobotGeometry/3(pitch)
  Torso Yaw [rad rad/s]/1 -> PositionUsingRobotGeometry/4(yaw)
  Torso Roll [rad rad/s]/1 -> PositionUsingRobotGeometry/2(roll)
  Right or Left [1/0]/1 -> PositionUsingRobotGeometry/1(right_left), [RightLeftPrimary]
  Right Leg Length [m m/s]/1 -> PositionUsingRobotGeometry/10(right_leg_length)
  Right Leg Roll [rad rad/s]/1 -> PositionUsingRobotGeometry/9(right_leg_lateral_angle)
  Right Leg Sagittal Angle [rad rad/s]/1 -> PositionUsingRobotGeometry/8(right_leg_sagittal_angle)
  Left Leg Length [m m/s]/1 -> PositionUsingRobotGeometry/7(left_leg_length)
  Left Leg Roll [rad rad/s]/1 -> PositionUsingRobotGeometry/6(left_leg_lateral_angle)
  Left Leg Sagittal Angle [rad rad/s]/1 -> PositionUsingRobotGeometry/5(left_leg_sagittal_angle)
  PositionUsingRobotGeometry/5(horizontal_com_position) -> Mux8/1
  " Acceleration Measurement [m/s^2] x3"/1 -> Kalman Filtering/11(COM XYZ Acceleration [m/s^2] x3), Demux2/1
  Demux2/3 -> Mux/3
  Demux2/1 -> Mux8/3
  Demux2/2 -> Mux9/3
  Mux3/1 -> Switch/3
  "[ddx, ddy, ddz]"/1 -> COM Acceleration [m/s^2] x3/1
  Mux8/1 -> Kalman Filtering/8("Initial [x, dx, ddx] [m, m/s, m/s^2]"), Demux5/1, Mux3/1
  Mux9/1 -> Kalman Filtering/9("Initial [y, dy, ddy] [m, m/s, m/s^2]"), Demux7/1, Mux3/2

== system vertical_smm_3d_with_xz_lqr_with_torque_cmds/Control/Behavior Control/Torque Distribution Left ==
  Leg Torque [Nm] : Inport
  Leg Force [N] : Inport  Port=2
  w [m] : Inport  Port=3
  Gain : Gain  Gain=0.5
  Gain1 : Gain  Gain=0.5
  Motor Torque Saturation Optimization : MATLAB Function  TreatAsAtomicUnit=on
  Product : Product  RndMeth=Zero
  Sum : Sum  Inputs=|++
  Sum1 : Sum  Inputs=+-|
  Back Torque [Nm] : Outport
  Front Torque [Nm] : Outport  Port=2
  wires:
  Gain/1 -> Motor Torque Saturation Optimization/1(x1s)
  Gain1/1 -> Motor Torque Saturation Optimization/2(x2s)
  Product/1 -> Gain1/1
  Leg Force [N]/1 -> Product/1
  Motor Torque Saturation Optimization/2(t2) -> Sum/2, Sum1/2
  w [m]/1 -> Product/2
  Motor Torque Saturation Optimization/1(t1) -> Sum1/1, Sum/1
  Sum/1 -> Front Torque [Nm]/1
  Leg Torque [Nm]/1 -> Gain/1
  Sum1/1 -> Back Torque [Nm]/1

== system vertical_smm_3d_with_xz_lqr_with_torque_cmds/Control/Behavior Control/Torque Distribution Right ==
  Leg Torque [Nm] : Inport
  Leg Force [N] : Inport  Port=2
  w [m] : Inport  Port=3
  Gain : Gain  Gain=0.5
  Gain1 : Gain  Gain=0.5
  Motor Torque Saturation Optimization : MATLAB Function  TreatAsAtomicUnit=on
  Product : Product  RndMeth=Zero
  Sum : Sum  Inputs=|++
  Sum1 : Sum  Inputs=+-|
  Back Torque [Nm] : Outport
  Front Torque [Nm] : Outport  Port=2
  wires:
  Sum1/1 -> Back Torque [Nm]/1
  Leg Torque [Nm]/1 -> Gain/1
  Sum/1 -> Front Torque [Nm]/1
  Motor Torque Saturation Optimization/1(t1) -> Sum/1, Sum1/1
  w [m]/1 -> Product/2
  Motor Torque Saturation Optimization/2(t2) -> Sum1/2, Sum/2
  Leg Force [N]/1 -> Product/1
  Product/1 -> Gain1/1
  Gain1/1 -> Motor Torque Saturation Optimization/2(x2s)
  Gain/1 -> Motor Torque Saturation Optimization/1(x1s)

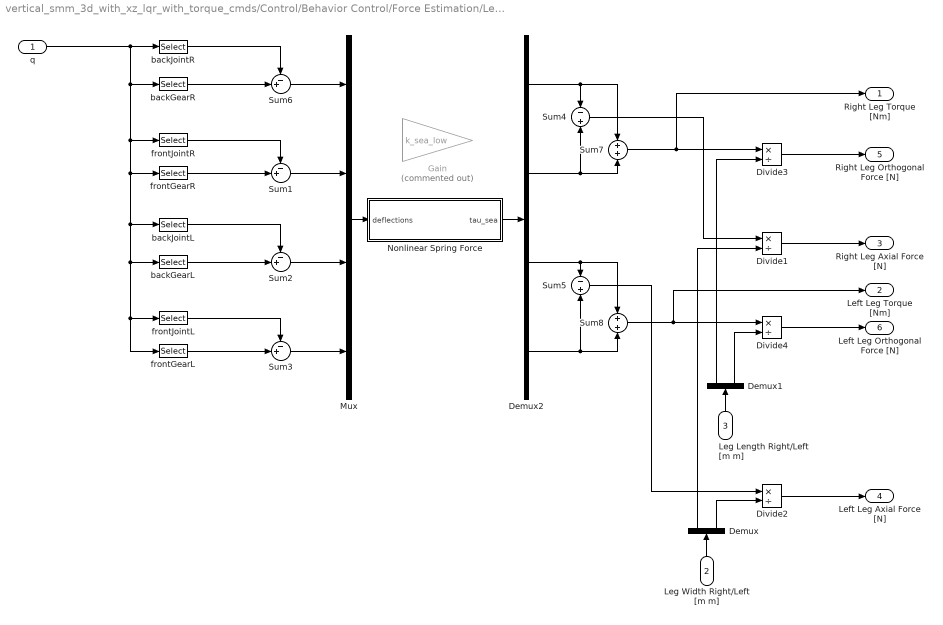
== system vertical_smm_3d_with_xz_lqr_with_torque_cmds/Control/Behavior Control/Force Estimation/Leg Force Measurements ==
  q : Inport
  Leg Width Right/Left [m m] : Inport  Port=2
  Leg Length Right/Left [m m] : Inport  Port=3
  Demux : Demux  Outputs=2
  Demux1 : Demux  Outputs=2
  Demux2 : Demux
  Divide{1..4} (4 alike) : Product  Inputs=*/
  Gain : Gain  Commented=on  Gain=k_sea_low
  Mux : Mux
  Nonlinear Spring Force : MATLAB Function  TreatAsAtomicUnit=on
  Sum{1..3,6} (4 alike) : Sum  Inputs=-+|
  Sum4 : Sum  Inputs=-|+
  Sum5 : Sum  Inputs=-|+
  Sum7 : Sum  Inputs=+|+
  Sum8 : Sum  Inputs=+|+
  backGearL : Selector  InputPortWidth=13  Indices=[6]
  backGearR : Selector  InputPortWidth=13  Indices=[2]
  backJointL : Selector  InputPortWidth=13  Indices=[5]
  backJointR : Selector  InputPortWidth=13  Indices=[1]
  frontGearL : Selector  InputPortWidth=13  Indices=[8]
  frontGearR : Selector  InputPortWidth=13  Indices=[4]
  frontJointL : Selector  InputPortWidth=13  Indices=[7]
  frontJointR : Selector  InputPortWidth=13  Indices=[3]
  Right Leg Torque [Nm] : Outport
  Left Leg Torque [Nm] : Outport  Port=2
  Right Leg Axial Force [N] : Outport  Port=3
  Left Leg Axial Force [N] : Outport  Port=4
  Right Leg Orthogonal Force [N] : Outport  Port=5
  Left Leg Orthogonal Force [N] : Outport  Port=6
  wires:
  Sum3/1 -> Mux/4
  Sum2/1 -> Mux/3
  backJointL/1 -> Sum2/1
  frontGearL/1 -> Sum3/2
  frontJointL/1 -> Sum3/1
  backGearL/1 -> Sum2/2
  Sum6/1 -> Mux/1
  Sum1/1 -> Mux/2
  backJointR/1 -> Sum6/1
  frontGearR/1 -> Sum1/2
  frontJointR/1 -> Sum1/1
  backGearR/1 -> Sum6/2
  q/1 -> backGearR/1, backJointL/1, frontJointL/1, frontGearL/1, backGearL/1, frontGearR/1, frontJointR/1, backJointR/1
  Demux2/1 -> Sum4/1, Sum7/1
  Demux2/2 -> Sum7/2, Sum4/2
  Demux2/4 -> Sum5/2, Sum8/2
  Sum4/1 -> Divide1/1
  Sum5/1 -> Divide2/1
  Leg Width Right/Left [m m]/1 -> Demux/1
  Demux/1 -> Divide1/2
  Demux/2 -> Divide2/2
  Divide1/1 -> Right Leg Axial Force [N]/1
  Divide2/1 -> Left Leg Axial Force [N]/1
  Demux2/3 -> Sum8/1, Sum5/1
  Sum7/1 -> Divide3/1, Right Leg Torque [Nm]/1
  Sum8/1 -> Divide4/1, Left Leg Torque [Nm]/1
  Demux1/1 -> Divide3/2
  Demux1/2 -> Divide4/2
  Leg Length Right/Left [m m]/1 -> Demux1/1
  Divide3/1 -> Right Leg Orthogonal Force [N]/1
  Divide4/1 -> Left Leg Orthogonal Force [N]/1
  Mux/1 -> Nonlinear Spring Force/1(deflections)
  Nonlinear Spring Force/1(tau_sea) -> Demux2/1

== system vertical_smm_3d_with_xz_lqr_with_torque_cmds/Control/Behavior Control/Force Estimation/Leg Plane GRF ==
  Axial Force [N] : Inport
  Orthogonal Force [N] : Inport  Port=2
  Torso Pitch [rad] : Inport  Port=3
  Leg Angle [rad] : Inport  Port=4
  Gain : Gain  Gain=-1
  Product : Product
  Product1 : Product
  Sum : Sum  Inputs=++|
  Sum1 : Sum  Inputs=+|+
  Trigonometric Function : Trigonometry  Operator=cos
  Trigonometric Function1 : Trigonometry
  Vertical Force [N] : Outport
  wires:
  Product1/1 -> Sum1/2
  Sum1/1 -> Vertical Force [N]/1
  Trigonometric Function1/1 -> Product1/2
  Orthogonal Force [N]/1 -> Product1/1
  Axial Force [N]/1 -> Product/1
  Leg Angle [rad]/1 -> Sum/2
  Torso Pitch [rad]/1 -> Sum/1
  Trigonometric Function/1 -> Product/2
  Product/1 -> Gain/1
  Sum/1 -> Trigonometric Function/1, Trigonometric Function1/1
  Gain/1 -> Sum1/1

== system vertical_smm_3d_with_xz_lqr_with_torque_cmds/Control/Behavior Control/Primary and Lateral Behavior/Circular Buffer ==
  Flight [1/0] : Inport
  Exiting Stance [1/0] : Inport  Port=2
  Hopping [1/0] : Inport  Port=3
  dX [m/s] : Inport  Port=4
  dY [m/s] : Inport  Port=5
  X Foot Correction [m] : Inport  Port=6
  Y Foot Correction [m] : Inport  Port=7
  target dX [m/s] : Inport  Port=8
  target dY [m/s] : Inport  Port=9
  Buffer : MATLAB Function  TreatAsAtomicUnit=on  SystemSampleTime=sample_time
  Buffer1 : MATLAB Function  TreatAsAtomicUnit=on  SystemSampleTime=sample_time
  Buffer2 : MATLAB Function  TreatAsAtomicUnit=on  SystemSampleTime=sample_time
  Buffer3 : MATLAB Function  TreatAsAtomicUnit=on  SystemSampleTime=sample_time
  Buffer4 : MATLAB Function  TreatAsAtomicUnit=on  SystemSampleTime=sample_time
  Buffer5 : MATLAB Function  TreatAsAtomicUnit=on  SystemSampleTime=sample_time
  Buffer6 : MATLAB Function  TreatAsAtomicUnit=on  SystemSampleTime=sample_time
  Buffer7 : MATLAB Function  TreatAsAtomicUnit=on  SystemSampleTime=sample_time
  Demux : Demux  Outputs=6
  Detect Decrease : simulink/Logic and Bit Operations/Detect Decrease  vinit=0.0  InputProcessing=Inherited  OutDataTypeStr=boolean
  Enabled on Touchdown : Subsystem  TreatAsAtomicUnit=on
  Logical Operator : Logic  AllPortsSameDT=off  OutDataTypeStr=boolean
  Mux : Mux  Inputs=6
  buffer size5 : Constant  Value=recorded_steps
  "dX Touchdown History " : Outport
  X Foot Correction History : Outport  Port=2
  dX Takeoff History : Outport  Port=3
  "dY Touchdown History " : Outport  Port=4
  Y Foot Correction History : Outport  Port=5
  dY Takeoff History : Outport  Port=6
  target dX History : Outport  Port=7
  target dY History : Outport  Port=8
  wires:
  Enabled on Touchdown/1(Out) -> Demux/1
  Mux/1 -> Enabled on Touchdown/1(In)
  Logical Operator/1 -> Detect Decrease/1
  Flight [1/0]/1 -> Logical Operator/2
  dX [m/s]/1 -> Mux/1, Buffer2/1(data)
  dY [m/s]/1 -> Mux/2, Buffer5/1(data)
  Hopping [1/0]/1 -> Logical Operator/1
  Exiting Stance [1/0]/1 -> Buffer5/2(trigger), Buffer2/2(trigger), Buffer3/2(trigger), Buffer1/2(trigger), Buffer4/2(trigger), Buffer6/2(trigger), Buffer7/2(trigger), Buffer/2(trigger)
  target dY [m/s]/1 -> Mux/6
  Demux/5 -> Buffer6/1(data)
  Demux/6 -> Buffer7/1(data)
  buffer size5/1 -> Buffer5/3(buffer_size), Buffer3/3(buffer_size), Buffer1/3(buffer_size), Buffer4/3(buffer_size), Buffer6/3(buffer_size), Buffer7/3(buffer_size), Buffer/3(buffer_size), Buffer2/3(buffer_size)
  Buffer7/1(buffer) -> target dY History/1
  Buffer6/1(buffer) -> target dX History/1
  target dX [m/s]/1 -> Mux/5
  Demux/4 -> Buffer4/1(data)
  Y Foot Correction [m]/1 -> Mux/4
  Buffer5/1(buffer) -> dY Takeoff History/1
  Demux/2 -> Buffer3/1(data)
  Buffer4/1(buffer) -> Y Foot Correction History/1
  Buffer3/1(buffer) -> "dY Touchdown History "/1
  X Foot Correction [m]/1 -> Mux/3
  Demux/3 -> Buffer1/1(data)
  Demux/1 -> Buffer/1(data)
  Buffer2/1(buffer) -> dX Takeoff History/1
  Buffer1/1(buffer) -> X Foot Correction History/1
  Detect Decrease/1 -> Enabled on Touchdown/Enable
  Buffer/1(buffer) -> "dX Touchdown History "/1
